simulink subsystem "state_transition_monitor"  (R2020a)
settings: Solver=VariableStepAuto  StartTime=0.0  StopTime=10.0  RelTol=1e-3
undefined symbols (not defined in the file): bool_inspection, misu_Ts, T_101, T_102, T_103, T_104, T_201, T_202
libraries: simulink x2
settings Model: Creator=andrea  LastModifiedBy=stefano

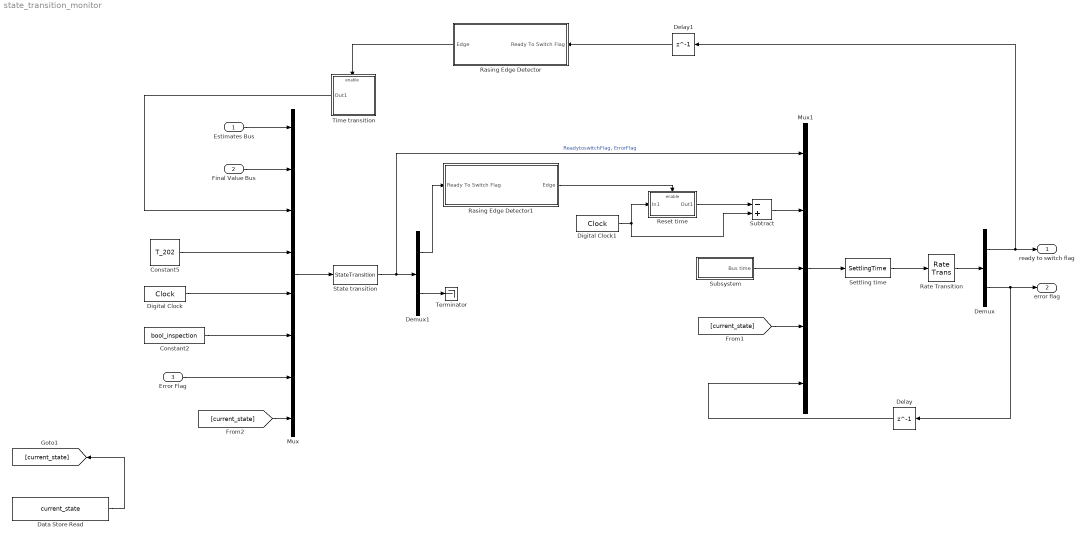
== system state_transition_monitor ==
  Estimates Bus : Inport
  Final Value Bus : Inport  Port=2
  Error Flag : Inport  Port=3
  Constant2 : Constant  Value=bool_inspection
  Constant5 : Constant  Value=T_202
  Data Store Read : DataStoreRead  DataStoreName=current_state
  Delay : Delay  DelayLength=1  SampleTime=misu_Ts
  Delay1 : Delay  DelayLength=1
  Demux : Demux  Outputs=2
  Demux1 : Demux  Outputs=2
  Digital Clock : DigitalClock  SampleTime=misu_Ts
  Digital Clock1 : DigitalClock  SampleTime=misu_Ts
  Mux : Mux  Inputs=8
  Mux1 : Mux  Inputs=5
  Rasing Edge Detector : Subsystem
  Rasing Edge Detector1 : Subsystem
  Rate Transition : RateTransition  Integrity=off  Deterministic=off  OutPortSampleTime=misu_Ts
  Reset time : Subsystem  TreatAsAtomicUnit=on
  "Settling time " : MATLABFcn  MATLABFcn=SettlingTime  OutputDimensions=2
  "State transition " : MATLABFcn  MATLABFcn=StateTransition  OutputDimensions=2
  Subsystem : Subsystem
  Subtract : Sum  Inputs=-+
  Terminator : Terminator
  Time transition : Subsystem
  ready to switch flag : Outport
  "error flag " : Outport  Port=2
  wires:
  [current_state] -> Mux1/4
  [current_state] -> Mux/8
  Data Store Read/1 -> [current_state]
  Time transition/1(Out1) -> Mux/3
  Rasing Edge Detector/1(Edge) -> Time transition/Enable
  Delay1/1 -> Rasing Edge Detector/1(Ready To Switch Flag)
  Demux1/2 -> Terminator/1
  Demux/2 -> Delay/1, "error flag "/1
  Subsystem/1("Bus time ") -> Mux1/3
  Mux1/1 -> "Settling time "/1
  Mux/1 -> "State transition "/1
  Subtract/1 -> Mux1/2
  Digital Clock1/1 -> Subtract/2, Reset time/1(In1)
  Reset time/1(Out1) -> Subtract/1
  "State transition "/1 -> Mux1/1, Demux1/1  "ReadytoswitchFlag, ErrorFlag"
  Demux1/1 -> Rasing Edge Detector1/1(Ready To Switch Flag)
  Rasing Edge Detector1/1(Edge) -> Reset time/Enable
  "Settling time "/1 -> Rate Transition/1
  Rate Transition/1 -> Demux/1
  Demux/1 -> ready to switch flag/1, Delay1/1
  Estimates Bus/1 -> Mux/1
  Final Value Bus/1 -> Mux/2
  Constant5/1 -> Mux/4
  Digital Clock/1 -> Mux/5
  Constant2/1 -> Mux/6
  Error Flag/1 -> Mux/7
  Delay/1 -> Mux1/5

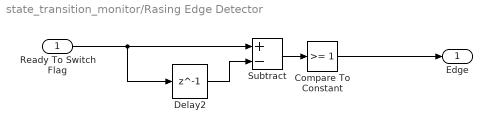
== system state_transition_monitor/Rasing Edge Detector ==
  Ready To Switch Flag : Inport
  Compare To Constant : simulink/Logic and Bit Operations/Compare To Constant  relop=>=  const=1  OutDataTypeStr=boolean
  Delay2 : Delay  DelayLength=1
  Subtract : Sum  Inputs=+-
  Edge : Outport
  wires:
  Ready To Switch Flag/1 -> Delay2/1, Subtract/1
  Compare To Constant/1 -> Edge/1
  Subtract/1 -> Compare To Constant/1
  Delay2/1 -> Subtract/2

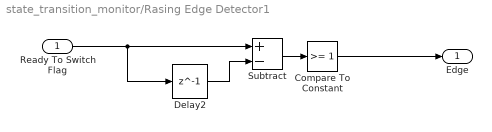
== system state_transition_monitor/Rasing Edge Detector1 ==
  Ready To Switch Flag : Inport
  Compare To Constant : simulink/Logic and Bit Operations/Compare To Constant  relop=>=  const=1  OutDataTypeStr=boolean
  Delay2 : Delay  DelayLength=1
  Subtract : Sum  Inputs=+-
  Edge : Outport
  wires:
  Ready To Switch Flag/1 -> Delay2/1, Subtract/1
  Compare To Constant/1 -> Edge/1
  Subtract/1 -> Compare To Constant/1
  Delay2/1 -> Subtract/2

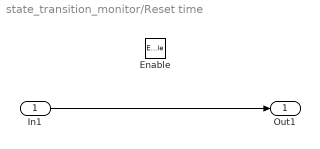
== system state_transition_monitor/Reset time ==
  In1 : Inport
  Enable : EnablePort
  Out1 : Outport
  wires:
  In1/1 -> Out1/1

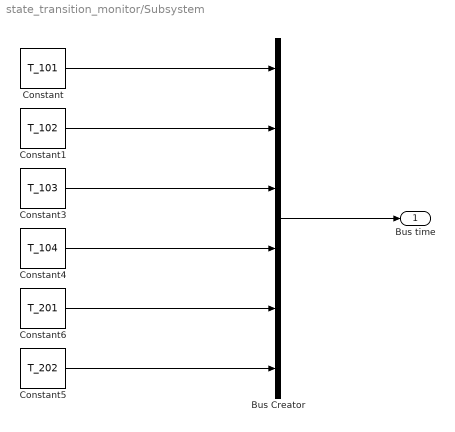
== system state_transition_monitor/Subsystem ==
  Bus Creator : BusCreator  Inputs=6
  Constant : Constant  Value=T_101
  Constant1 : Constant  Value=T_102
  Constant3 : Constant  Value=T_103
  Constant4 : Constant  Value=T_104
  Constant5 : Constant  Value=T_202
  Constant6 : Constant  Value=T_201
  "Bus time " : Outport
  wires:
  Constant/1 -> Bus Creator/1
  Constant1/1 -> Bus Creator/2
  Constant3/1 -> Bus Creator/3
  Constant4/1 -> Bus Creator/4
  Constant6/1 -> Bus Creator/5
  Constant5/1 -> Bus Creator/6
  Bus Creator/1 -> "Bus time "/1

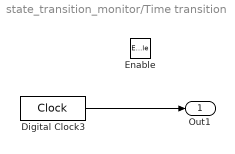
== system state_transition_monitor/Time transition ==
  Enable : EnablePort
  Digital Clock3 : DigitalClock  SampleTime=misu_Ts
  Out1 : Outport
  wires:
  Digital Clock3/1 -> Out1/1
